simulink model "HinfTenzo"  (R2015a)
settings: Solver=ode23  StartTime=0.0  StopTime=10  RelTol=1e-3
values from neighbouring files (symbols this model uses):
  A0 = tenzo_min_nominale.a    [HTenzoV10.m]    (also in HTenzoV11.m; HTenzoV12.m; HTenzoV13.m; HTenzoV14.m)
  amplitudeNoise = 2    [HTenzoV10.m]    (also in HTenzoV11.m; HTenzoV12.m; HTenzoV13.m; HTenzoV14.m)
  amplitudePertIN = 0    [HTenzoV10.m]    (also in HTenzoV11.m; HTenzoV12.m; HTenzoV13.m; HTenzoV14.m)
  amplitudePertOutptp = 0    [HTenzoV10.m]    (also in HTenzoV11.m; HTenzoV12.m; HTenzoV13.m; HTenzoV14.m)
  amplitudePertOutZ = 0    [HTenzoV10.m]    (also in HTenzoV11.m; HTenzoV12.m; HTenzoV13.m; HTenzoV14.m)
  B0 = tenzo_min_nominale.b    [HTenzoV10.m]    (also in HTenzoV11.m; HTenzoV12.m; HTenzoV13.m; HTenzoV14.m)
  C0 = tenzo_min_nominale.c    [HTenzoV10.m]    (also in HTenzoV11.m; HTenzoV12.m; HTenzoV13.m; HTenzoV14.m)
  cstPertIn = 0    [HTenzoV10.m]    (also in HTenzoV11.m; HTenzoV12.m; HTenzoV13.m; HTenzoV14.m)
  cstPertOut = 0    [HTenzoV10.m]    (also in HTenzoV11.m; HTenzoV12.m; HTenzoV13.m; HTenzoV14.m)
  D0 = tenzo_min_nominale.d    [HTenzoV10.m]    (also in HTenzoV11.m; HTenzoV12.m; HTenzoV13.m; HTenzoV14.m)
  Kinf = K123    [HTenzoV10.m]    (also in HTenzoV11.m; HTenzoV12.m; HTenzoV13.m; HTenzoV14.m)
  omegaNoise = 370    [HTenzoV10.m]    (also in HTenzoV11.m; HTenzoV12.m; HTenzoV13.m; HTenzoV14.m)
  omegaPertIN = 6    [HTenzoV10.m]    (also in HTenzoV11.m; HTenzoV12.m; HTenzoV13.m; HTenzoV14.m)
  omegaPertOut = 0.1    [HTenzoV10.m]    (also in HTenzoV11.m; HTenzoV12.m; HTenzoV13.m; HTenzoV14.m)
  randomAmpNoise = 1    [HTenzoV10.m]    (also in HTenzoV11.m; HTenzoV12.m; HTenzoV13.m; HTenzoV14.m)
undefined symbols (not defined in the file or in its folder): sigbuilder_block
settings Model: SimulationMode=rapid-accelerator  Creator=danilo  LastModifiedBy=userk
settings OptimizationCC: ExpressionDepthLimit=2147483647
settings DebuggingCC: UnderspecifiedInitializationDetection=Classic  MergeDetectMultiDrivingBlocksExec=none  SolverPrmCheckMsg=warning  FcnCallInpInsideContextMsg=UseLocalSettings  StateNameClashWarn=warning
settings GRTTargetCC: CombineOutputUpdateFcns=off  GRTInterface=on

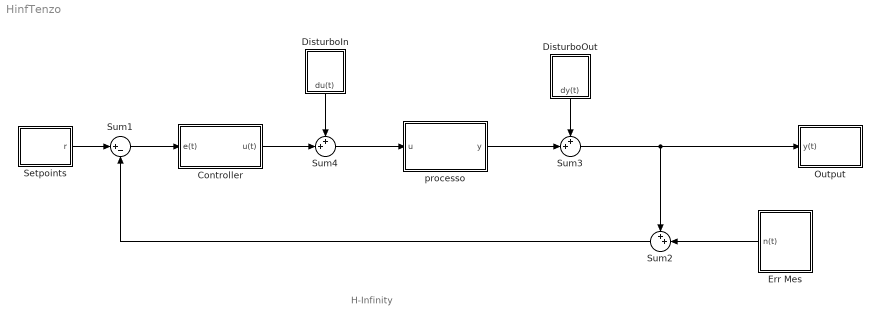
== system HinfTenzo ==
  note: H-Infinity
  Controller : Subsystem
  DisturboIn : Subsystem
  DisturboOut : Subsystem
  Err Mes : Subsystem
  Output : Subsystem
  Setpoints : Subsystem
  Sum1 : Sum  Inputs=|+-
  Sum2 : Sum  Inputs=++|
  Sum3 : Sum  Inputs=++|
  Sum4 : Sum  Inputs=++|
  processo : Subsystem
  wires:
  Sum2/1 -> Sum1/2
  Setpoints/1(r) -> Sum1/1
  Err Mes/1(n(t)) -> Sum2/2
  processo/1(y) -> Sum3/2
  DisturboIn/1(du(t)) -> Sum4/1
  Sum3/1 -> Sum2/1, Output/1(y(t))
  DisturboOut/1("dy(t) ") -> Sum3/1
  Sum4/1 -> processo/1(u)
  Sum1/1 -> Controller/1(e(t))
  Controller/1(u(t)) -> Sum4/2

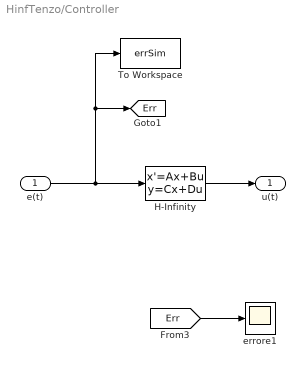
== system HinfTenzo/Controller ==
  e(t) : Inport
  H-Infinity : StateSpace  A=Kinf.a  B=Kinf.b  C=Kinf.c  D=Kinf.d  X0=0
  To Workspace : ToWorkspace  VariableName=errSim  SaveFormat=Structure  SampleTime=-1
  errore1 : Scope
      settings: ShowLegends=on  YMin=-12  YMax=1  SaveName=ScopeData8
  u(t) : Outport
  tag scope: Err=global
  wires:
  [Err] -> errore1/1
  e(t)/1 -> H-Infinity/1, To Workspace/1, [Err]
  H-Infinity/1 -> u(t)/1

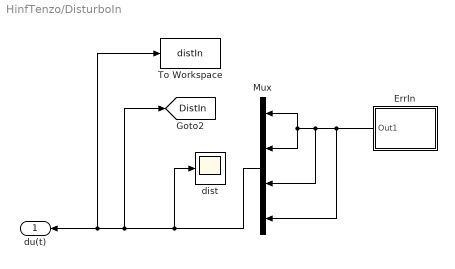
== system HinfTenzo/DisturboIn ==
  ErrIn : Subsystem
  Mux : Mux  Inputs=[1 1 1 1]
  To Workspace : ToWorkspace  VariableName=distIn  SaveFormat=Timeseries  SampleTime=-1
  dist : Scope
      settings: YMin=-700  YMax=150  SaveName=ScopeData5
  du(t) : Outport
  tag scope: DistIn=global
  wires:
  Mux/1 -> dist/1, [DistIn], To Workspace/1, du(t)/1
  ErrIn/1(Out1) -> Mux/4, Mux/3, Mux/2, Mux/1

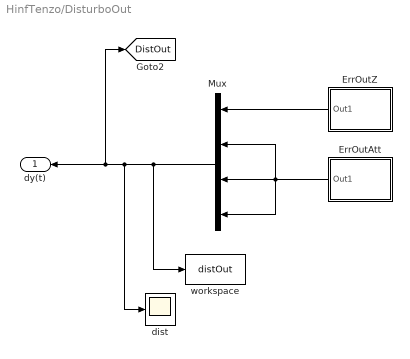
== system HinfTenzo/DisturboOut ==
  ErrOutAtt : Subsystem
  ErrOutZ : Subsystem
  Mux : Mux  Inputs=[1 1 1 1]
  dist : Scope
      settings: YMin=1  YMax=23  SaveName=ScopeData5
  "workspace " : ToWorkspace  VariableName=distOut  SaveFormat=Timeseries  SampleTime=-1
  "dy(t) " : Outport
  tag scope: DistOut=global
  wires:
  ErrOutZ/1(Out1) -> Mux/1
  ErrOutAtt/1(Out1) -> Mux/4, Mux/3, Mux/2
  Mux/1 -> "workspace "/1, dist/1, "dy(t) "/1, [DistOut]

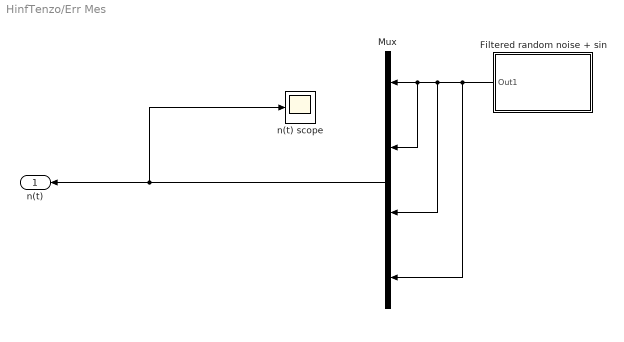
== system HinfTenzo/Err Mes ==
  Filtered random noise + sin : Subsystem
  Mux : Mux  Inputs=[1 1 1 1]
  n(t) scope : Scope
      settings: YMin=-0.08  YMax=0.02  SaveName=ScopeData21
  n(t) : Outport
  wires:
  Filtered random noise + sin/1(Out1) -> Mux/4, Mux/3, Mux/2, Mux/1
  Mux/1 -> n(t) scope/1, n(t)/1

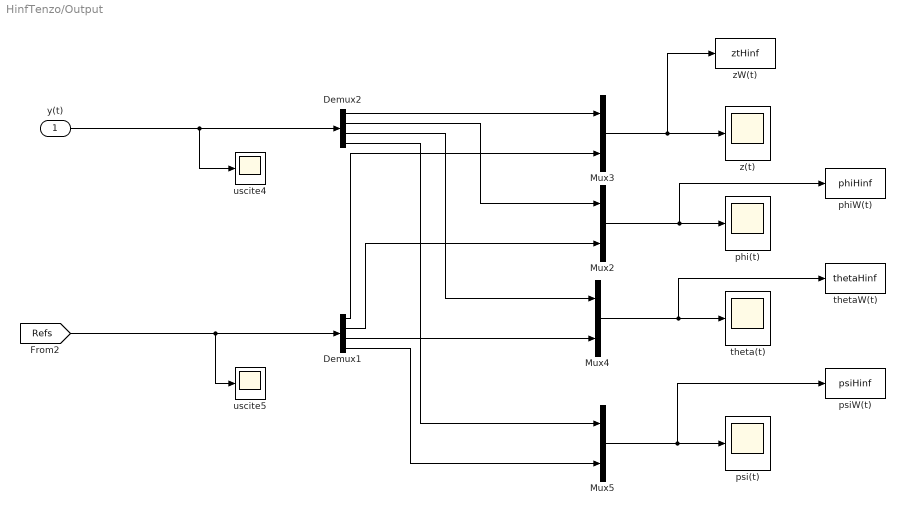
== system HinfTenzo/Output ==
  y(t) : Inport
  Demux1 : Demux
  Demux2 : Demux
  Mux{2..5} (4 alike) : Mux  Inputs=2
  phi(t) : Scope
      settings: TickLabels=on  ShowLegends=on  TimeRange=10  YMin=-25  YMax=55  SaveName=ScopeData4
  phiW(t) : ToWorkspace  VariableName=phiHinf  SaveFormat=Timeseries  SampleTime=-1
  psi(t) : Scope
      settings: TickLabels=on  ShowLegends=on  YMin=-0.0525  YMax=0  SaveName=ScopeData7
  psiW(t) : ToWorkspace  VariableName=psiHinf  SaveFormat=Timeseries  SampleTime=-1
  theta(t) : Scope
      settings: TickLabels=on  ShowLegends=on  YMin=-275  YMax=275  SaveName=ScopeData6
  thetaW(t) : ToWorkspace  VariableName=thetaHinf  SaveFormat=Timeseries  SampleTime=-1
  uscite4 : Scope
      settings: ShowLegends=on  YMin=675  YMax=975  SaveName=ScopeData2
  uscite5 : Scope
      settings: ShowLegends=on  YMin=-50  YMax=200  SaveName=ScopeData9
  z(t) : Scope
      settings: TickLabels=on  ShowLegends=on  YMin=3  YMax=10
  zW(t) : ToWorkspace  VariableName=ztHinf  SaveFormat=Timeseries  SampleTime=-1
  wires:
  [Refs] -> Demux1/1, uscite5/1
  Demux1/1 -> Mux3/2
  Mux2/1 -> phiW(t)/1, phi(t)/1
  Demux2/2 -> Mux2/1
  Mux3/1 -> zW(t)/1, z(t)/1
  Demux2/1 -> Mux3/1
  Mux4/1 -> thetaW(t)/1, theta(t)/1
  Demux2/3 -> Mux4/1
  Mux5/1 -> psiW(t)/1, psi(t)/1
  Demux2/4 -> Mux5/1
  Demux1/2 -> Mux2/2
  Demux1/3 -> Mux4/2
  Demux1/4 -> Mux5/2
  y(t)/1 -> Demux2/1, uscite4/1

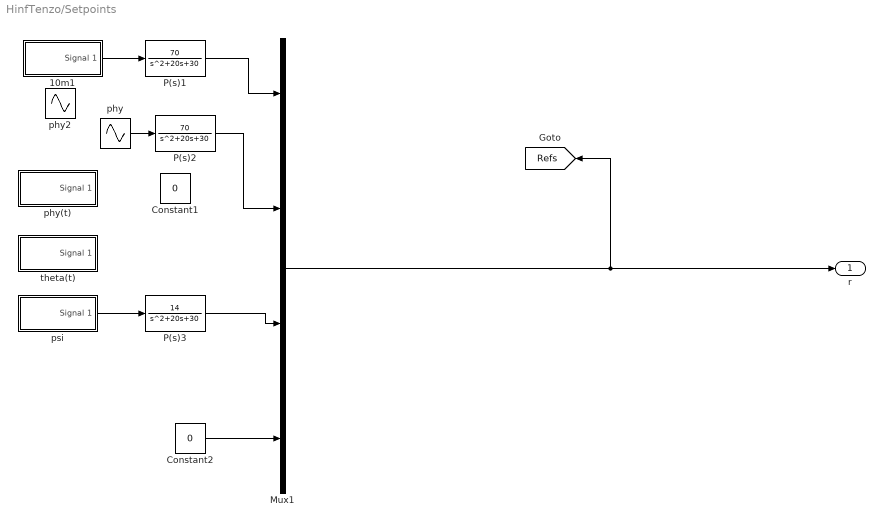
== system HinfTenzo/Setpoints ==
  10m1 : Subsystem  Tag=STV Subsys  LoadFcn=sigbuilder_block('load');  StartFcn=sigbuilder_block('start');  StopFcn=sigbuilder_block('stop');  ClipboardFcn=sigbuilder_block('clipboard');  mask(Sigbuilder block){}
      mask help: Simulink:masks:SigbuilderBlock_MD
      mask init:
      | if ~strcmp(get_param(bdroot(gcbh),'SimulationStatus'),'stopped') tuvar = sigbuilder_block('maskInit'); end
      settings: CopyFcn=sigbuilder_block('copy');  DeleteFcn=sigbuilder_block('delete');  ModelCloseFcn=sigbuilder_block('modelClose');  PreSaveFcn=sigbuilder_block('preSave');  PauseFcn=sigbuilder_block('pause');  ContinueFcn=sigbuilder_block('continue');  NameChangeFcn=sigbuilder_block('namechange');  OpenFcn=sigbuilder_block('open',[341.6 120.8 550.4 400 ]);  CloseFcn=sigbuilder_block('close');
      mask Display: plot(0, 0, 100, 100,[2, 2, 32, 32, 2], [68, 8, 8, 68, 68],[32, 2], [38, 38], [32, 19, 2],[53, 60, 44], [32, 17, 17, 2],[16, 16, 31, 31]);txt = getActiveGroup(gcbh);text(2, 100, txt,'verticalAlignment', 'top');
  Constant1 : Constant  Value=0
  Constant2 : Constant  Value=0
  Mux1 : Mux  Inputs=[1 1 1 1]
  P(s)1 : TransferFcn  Numerator=70  Denominator=[1 20 30]
  P(s)2 : TransferFcn  Numerator=70  Denominator=[1 20 30]
  P(s)3 : TransferFcn  Numerator=14  Denominator=[1 20 30]
  phy : Sin  Amplitude=50  SampleTime=0
  phy(t) : Subsystem  Tag=STV Subsys  LoadFcn=sigbuilder_block('load');  StartFcn=sigbuilder_block('start');  StopFcn=sigbuilder_block('stop');  ClipboardFcn=sigbuilder_block('clipboard');  mask(Sigbuilder block){}
      mask help: Simulink:masks:SigbuilderBlock_MD
      mask init:
      | if ~strcmp(get_param(bdroot(gcbh),'SimulationStatus'),'stopped') tuvar = sigbuilder_block('maskInit'); end
      settings: CopyFcn=sigbuilder_block('copy');  DeleteFcn=sigbuilder_block('delete');  ModelCloseFcn=sigbuilder_block('modelClose');  PreSaveFcn=sigbuilder_block('preSave');  PauseFcn=sigbuilder_block('pause');  ContinueFcn=sigbuilder_block('continue');  NameChangeFcn=sigbuilder_block('namechange');  OpenFcn=sigbuilder_block('open',[341.6 120.8 550.4 400 ]);  CloseFcn=sigbuilder_block('close');
      mask Display: plot(0, 0, 100, 100,[2, 2, 32, 32, 2], [68, 8, 8, 68, 68],[32, 2], [38, 38], [32, 19, 2],[53, 60, 44], [32, 17, 17, 2],[16, 16, 31, 31]);txt = getActiveGroup(gcbh);text(2, 100, txt,'verticalAlignment', 'top');
  phy2 : Sin  Amplitude=10  Frequency=0.2  SampleTime=0
  "psi " : Subsystem  Tag=STV Subsys  LoadFcn=sigbuilder_block('load');  StartFcn=sigbuilder_block('start');  StopFcn=sigbuilder_block('stop');  ClipboardFcn=sigbuilder_block('clipboard');  mask(Sigbuilder block){}
      mask help: Simulink:masks:SigbuilderBlock_MD
      mask init:
      | if ~strcmp(get_param(bdroot(gcbh),'SimulationStatus'),'stopped') tuvar = sigbuilder_block('maskInit'); end
      settings: CopyFcn=sigbuilder_block('copy');  DeleteFcn=sigbuilder_block('delete');  ModelCloseFcn=sigbuilder_block('modelClose');  PreSaveFcn=sigbuilder_block('preSave');  PauseFcn=sigbuilder_block('pause');  ContinueFcn=sigbuilder_block('continue');  NameChangeFcn=sigbuilder_block('namechange');  OpenFcn=sigbuilder_block('open',[341.6 120.8 550.4 400 ]);  CloseFcn=sigbuilder_block('close');
      mask Display: plot(0, 0, 100, 100,[2, 2, 32, 32, 2], [68, 8, 8, 68, 68],[32, 2], [38, 38], [32, 19, 2],[53, 60, 44], [32, 17, 17, 2],[16, 16, 31, 31]);txt = getActiveGroup(gcbh);text(2, 100, txt,'verticalAlignment', 'top');
  theta(t) : Subsystem  Tag=STV Subsys  LoadFcn=sigbuilder_block('load');  StartFcn=sigbuilder_block('start');  StopFcn=sigbuilder_block('stop');  ClipboardFcn=sigbuilder_block('clipboard');  mask(Sigbuilder block){}
      mask help: Simulink:masks:SigbuilderBlock_MD
      mask init:
      | if ~strcmp(get_param(bdroot(gcbh),'SimulationStatus'),'stopped') tuvar = sigbuilder_block('maskInit'); end
      settings: CopyFcn=sigbuilder_block('copy');  DeleteFcn=sigbuilder_block('delete');  ModelCloseFcn=sigbuilder_block('modelClose');  PreSaveFcn=sigbuilder_block('preSave');  PauseFcn=sigbuilder_block('pause');  ContinueFcn=sigbuilder_block('continue');  NameChangeFcn=sigbuilder_block('namechange');  OpenFcn=sigbuilder_block('open',[341.6 120.8 550.4 400 ]);  CloseFcn=sigbuilder_block('close');
      mask Display: plot(0, 0, 100, 100,[2, 2, 32, 32, 2], [68, 8, 8, 68, 68],[32, 2], [38, 38], [32, 19, 2],[53, 60, 44], [32, 17, 17, 2],[16, 16, 31, 31]);txt = getActiveGroup(gcbh);text(2, 100, txt,'verticalAlignment', 'top');
  r : Outport
  tag scope: Refs=global
  wires:
  10m1/1(Signal 1) -> P(s)1/1
  phy/1 -> P(s)2/1
  Constant2/1 -> Mux1/4
  "psi "/1(Signal 1) -> P(s)3/1
  Mux1/1 -> [Refs], r/1
  P(s)1/1 -> Mux1/1
  P(s)2/1 -> Mux1/2
  P(s)3/1 -> Mux1/3

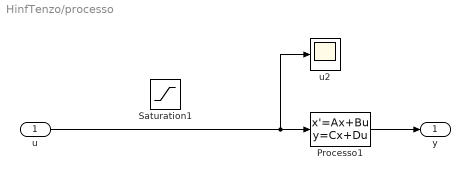
== system HinfTenzo/processo ==
  u : Inport
  Processo1 : StateSpace  A=A0  B=B0  C=C0  D=D0  X0=0
  Saturation1 : Saturate  UpperLimit=17000  LowerLimit=-17000
  u2 : Scope
      settings: TimeRange=10  YMin=-70000  YMax=80000  SaveName=ScopeData10
  y : Outport
  wires:
  Processo1/1 -> y/1
  u/1 -> u2/1, Processo1/1

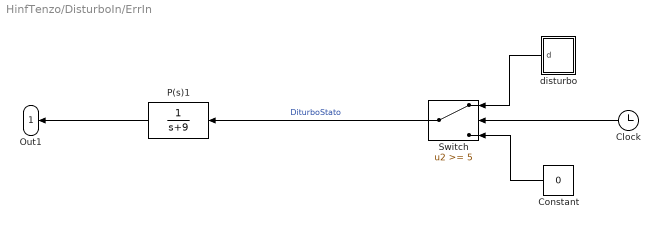
== system HinfTenzo/DisturboIn/ErrIn ==
  Clock : Clock
  Constant : Constant  Value=0
  P(s)1 : TransferFcn  Numerator=1  Denominator=[1 9]
  Switch : Switch  Threshold=5
  disturbo : Subsystem
  Out1 : Outport
  wires:
  Constant/1 -> Switch/3
  disturbo/1(d) -> Switch/1
  Switch/1 -> P(s)1/1  "DiturboStato"
  Clock/1 -> Switch/2
  P(s)1/1 -> Out1/1

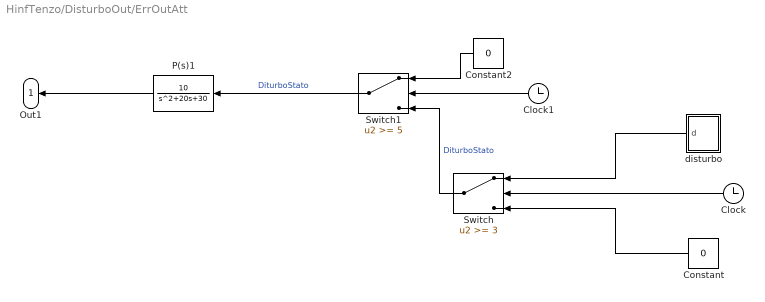
== system HinfTenzo/DisturboOut/ErrOutAtt ==
  Clock : Clock
  Clock1 : Clock
  Constant : Constant  Value=0
  Constant2 : Constant  Value=0
  P(s)1 : TransferFcn  Numerator=10  Denominator=[1 20 30]
  Switch : Switch  Threshold=3
  Switch1 : Switch  Threshold=5
  disturbo : Subsystem
  Out1 : Outport
  wires:
  P(s)1/1 -> Out1/1
  Switch1/1 -> P(s)1/1  "DiturboStato"
  Clock1/1 -> Switch1/2
  Constant2/1 -> Switch1/1
  Constant/1 -> Switch/3
  Switch/1 -> Switch1/3  "DiturboStato"
  Clock/1 -> Switch/2
  disturbo/1(d) -> Switch/1

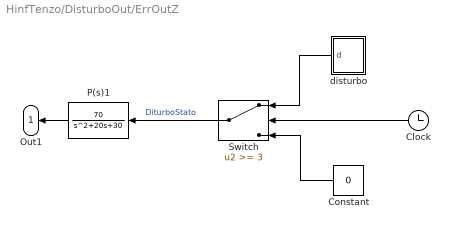
== system HinfTenzo/DisturboOut/ErrOutZ ==
  Clock : Clock
  Constant : Constant  Value=0
  P(s)1 : TransferFcn  Numerator=70  Denominator=[1 20 30]
  Switch : Switch  Threshold=3
  disturbo : Subsystem
  Out1 : Outport
  wires:
  Clock/1 -> Switch/2
  Switch/1 -> P(s)1/1  "DiturboStato"
  disturbo/1(d) -> Switch/1
  Constant/1 -> Switch/3
  P(s)1/1 -> Out1/1

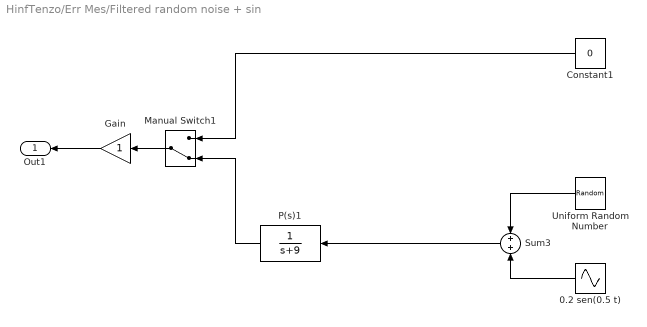
== system HinfTenzo/Err Mes/Filtered random noise + sin ==
  0.2 sen(0.5 t) : Sin  Amplitude=amplitudeNoise  Frequency=omegaNoise  Phase=1  SampleTime=0
  Constant1 : Constant  Value=0
  Gain : Gain
  Manual Switch1 : ManualSwitch  CurrentSetting=0
  P(s)1 : TransferFcn  Numerator=1  Denominator=[1 9]
  Sum3 : Sum
  Uniform Random Number : UniformRandomNumber  Minimum=-randomAmpNoise  Maximum=randomAmpNoise  SampleTime=0.1
  Out1 : Outport
  wires:
  Uniform Random Number/1 -> Sum3/1
  Constant1/1 -> Manual Switch1/1
  Sum3/1 -> P(s)1/1
  Gain/1 -> Out1/1
  P(s)1/1 -> Manual Switch1/2
  Manual Switch1/1 -> Gain/1
  0.2 sen(0.5 t)/1 -> Sum3/2

== system HinfTenzo/Setpoints/10m1 ==
  Demux : Demux  Tag=STV Demux  Outputs=1
  FromWs : FromWorkspace  Tag=STV FromWs  VariableName=tuvar  SampleTime=0
      SigBuilderData=|
      | common.afterFinalStr = 'Extrapolate'
      | common.sampleTime = 0
      | dataSet.timeRange = [0 10]
      | dataSet.name = 'Group 1'
      | sbobj.Groups.Name = 'Group 1'
      | sbobj.Groups.Signals.Name = 'Signal 1'
      | sbobj.Groups.Signals.XData = [0 3 7 10]
      | sbobj.Groups.Signals.YData = [0 10 10 0]
  Signal 1 : Outport  Tag=STV Outport
  wires:
  FromWs/1 -> Demux/1
  Demux/1 -> Signal 1/1

== system HinfTenzo/Setpoints/phy(t) ==
  Demux : Demux  Tag=STV Demux  Outputs=1
  FromWs : FromWorkspace  Tag=STV FromWs  VariableName=tuvar  SampleTime=0
      SigBuilderData=|
      | common.afterFinalStr = 'Extrapolate'
      | common.sampleTime = 0
      | dataSet.timeRange = [0 10]
      | dataSet.name = 'Group 1'
      | sbobj.Groups.Name = 'Group 1'
      | sbobj.Groups.Signals.Name = 'Signal 1'
      | sbobj.Groups.Signals.XData = [0 0.98 2 2 10]
      | sbobj.Groups.Signals.YData = [0 0 50 0 0]
  Signal 1 : Outport  Tag=STV Outport
  wires:
  FromWs/1 -> Demux/1
  Demux/1 -> Signal 1/1

== system HinfTenzo/Setpoints/psi  ==
  Demux : Demux  Tag=STV Demux  Outputs=1
  FromWs : FromWorkspace  Tag=STV FromWs  VariableName=tuvar  SampleTime=0
      SigBuilderData=|
      | common.afterFinalStr = 'Extrapolate'
      | common.sampleTime = 0
      | dataSet.timeRange = [0 10]
      | dataSet.name = 'Group 1'
      | sbobj.Groups.Name = 'Group 1'
      | sbobj.Groups.Signals.Name = 'Signal 1'
      | sbobj.Groups.Signals.XData = [0 4.06 6.82 10]
      | sbobj.Groups.Signals.YData = [0 190 0 0]
  Signal 1 : Outport  Tag=STV Outport
  wires:
  FromWs/1 -> Demux/1
  Demux/1 -> Signal 1/1

== system HinfTenzo/Setpoints/theta(t) ==
  Demux : Demux  Tag=STV Demux  Outputs=1
  FromWs : FromWorkspace  Tag=STV FromWs  VariableName=tuvar  SampleTime=0
      SigBuilderData=|
      | common.afterFinalStr = 'Extrapolate'
      | common.sampleTime = 0
      | dataSet.timeRange = [0 10]
      | dataSet.name = 'Group 1'
      | sbobj.Groups.Name = 'Group 1'
      | sbobj.Groups.Signals.Name = 'Signal 1'
      | sbobj.Groups.Signals.XData = [0 4.06 6.82 6.82 10]
      | sbobj.Groups.Signals.YData = [0 0 20 0 0]
  Signal 1 : Outport  Tag=STV Outport
  wires:
  FromWs/1 -> Demux/1
  Demux/1 -> Signal 1/1

== system HinfTenzo/DisturboIn/ErrIn/disturbo ==
  Constant : Constant  Value=cstPertIn
  SineIn : Sin  Amplitude=amplitudePertIN  Frequency=omegaPertIN  SampleTime=0
  Sum2 : Sum  Inputs=|++
  d : Outport
  wires:
  Sum2/1 -> d/1
  Constant/1 -> Sum2/1
  SineIn/1 -> Sum2/2

== system HinfTenzo/DisturboOut/ErrOutAtt/disturbo ==
  Constant : Constant  Value=cstPertOut
  SineOut : Sin  Amplitude=amplitudePertOutptp  Frequency=omegaPertOut  SampleTime=0
  Sum2 : Sum  Inputs=|++
  d : Outport
  wires:
  Sum2/1 -> d/1
  Constant/1 -> Sum2/1
  SineOut/1 -> Sum2/2

== system HinfTenzo/DisturboOut/ErrOutZ/disturbo ==
  Constant : Constant  Value=cstPertOut
  SineOut : Sin  Amplitude=amplitudePertOutZ  Frequency=omegaPertOut  SampleTime=0
  Sum2 : Sum  Inputs=|++
  d : Outport
  wires:
  SineOut/1 -> Sum2/2
  Constant/1 -> Sum2/1
  Sum2/1 -> d/1
